simulink model "payment_donation_hcs_2020"  (R2020a)
settings: Solver=VariableStepAuto  StartTime=0.0  StopTime=10.0  RelTol=1e-3
(part 2 of 2)

== system payment_donation_hcs_2020/F_B9 ==
  FB : Inport
      mask Display:
      | plot([0 60-10],[0 0]);
      | plot([0 0],[0 16]);
      | plot([0 60-10],[16 16]);
      | plot([60-10 60],[16 8]);
      | plot([60-10 60],[0 8]);
  Ground : Ground
  Terminator : Terminator
  CA : Outport
      mask Display:
      | plot([10 65],[0 0]);
      | plot([65-1 65-1],[0 16]);
      | plot([10 65],[16 16]);
      | plot([0 10],[8 16]);
      | plot([0 10],[8 0]);
  wires:
  FB/1 -> Terminator/1
  Ground/1 -> CA/1

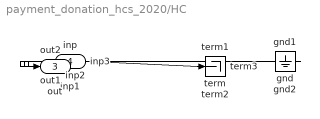
== system payment_donation_hcs_2020/HC ==
  inp : Inport
  inp1 : Inport  Port=2
  inp2 : Inport  Port=3
  inp3 : Inport  Port=4
  gnd : Ground
  gnd1 : Ground
  gnd2 : Ground
  term{,1..3} (4 alike) : Terminator
  out1 : Outport
  out2 : Outport  Port=2
  out : Outport  Port=3
  wires:
  inp/1 -> term/1
  gnd1/1 -> out1/1
  gnd2/1 -> out2/1
  gnd/1 -> out/1
  inp1/1 -> term1/1
  inp2/1 -> term2/1
  inp3/1 -> term3/1

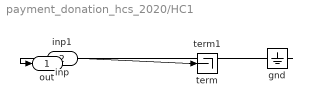
== system payment_donation_hcs_2020/HC1 ==
  inp : Inport
  inp1 : Inport  Port=2
  gnd : Ground
  term : Terminator
  term1 : Terminator
  out : Outport
  wires:
  inp/1 -> term/1
  gnd/1 -> out/1
  inp1/1 -> term1/1
